simulink model "TVC_Model"  (R2019a)
settings: Solver=FixedStepAuto  StartTime=0.0  StopTime=ENV.t_f  FixedStep=.01  MaxStep=.01  RelTol=1e-3  EnableMultiTasking=on
undefined symbols (not defined in the file or in its folder): ACT, CTRL, ENV, Motor, VEH
libraries: Force_Moment_Sublibrary x4, Rail_UL x1, Environment_UL x1, Launch_Vehicle_CL x1
settings Model: ExtModeTrigDuration=2  Creator=John Jr  LastModifiedBy=John Jr
settings SolverCC: MaxConsecutiveMinStep=5
settings DataIOCC: LimitDataPoints=on  SaveFinalState=on  ReturnWorkspaceOutputs=off
settings OptimizationCC: DefaultParameterBehavior=Inlined  MaxStackSize=64
settings DebuggingCC: AllowSymbolicDim=off  SFUnexpectedBacktrackingDiag=warning  SFNoUnconditionalDefaultTransitionDiag=warning  SFExecutionAtInitializationDiag=none  ArithmeticOperatorsInVariantConditions=warning
settings HardwareCC: ProdBitPerInt=16  ProdBitPerPointer=16  ProdBitPerSizeT=16  ProdBitPerPtrDiffT=16  ProdLargestAtomicFloat=None  ProdWordSize=8  ProdHWDeviceType=Atmel->AVR  UseEmbeddedCoderFeatures=off  UseSimulinkCoderFeatures=off
settings ModelReferenceCC: PropagateSignalLabelsOutOfModel=off
settings SFSimCC: SimUseLocalCustomCode=off  MATLABDynamicMemAlloc=off
settings RTWCC: Description=Generic Real-Time Target  RTWUseLocalCustomCode=off  Toolchain=Microsoft Visual C++ 2019 v16.0 | nmake (64-bit Windows)  BuildConfiguration=Faster Runs
settings CodeAppCC: StateflowObjectComments=on
settings GRTTargetCC: TargetLangStandard=C89/C90 (ANSI)
settings ConfigComp: CovMetricSettings=dw  CovHtmlReporting=on  CovSaveCumulativeToWorkspaceVar=on  CovSaveSingleToWorkspaceVar=on  CovExternalEMLEnable=off

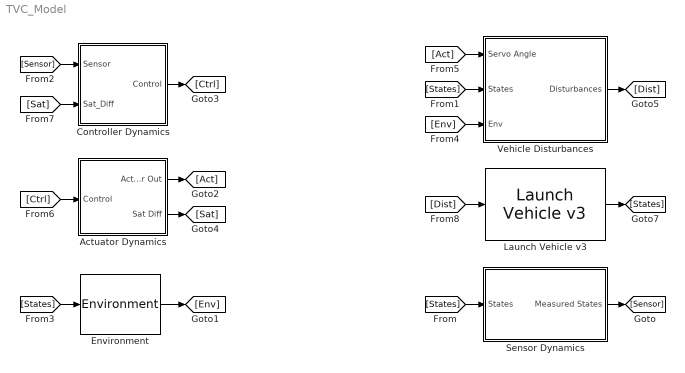
== system TVC_Model ==
  Actuator Dynamics : Subsystem
  Controller Dynamics : Subsystem
  Environment : Environment_UL/Environment  g=ENV.g  rho_b=ENV.rho_b  z_0=ENV.z_0  T=ENV.T  M=ENV.M  R=ENV.R  v_w0=ENV.v_w0  v_wf=ENV.v_wf
  Launch Vehicle v3 : Launch_Vehicle_CL/Launch Vehicle v3  SystemSampleTime=-1
  Sensor Dynamics : Subsystem
  Vehicle Disturbances : Subsystem
  wires:
  Launch Vehicle v3/1 -> [States]
  [States] -> Sensor Dynamics/1(States)
  [States] -> Vehicle Disturbances/2(States)
  Sensor Dynamics/1(Measured States) -> [Sensor]
  [Sensor] -> Controller Dynamics/1(Sensor)
  [States] -> Environment/1
  Environment/1 -> [Env]
  [Env] -> Vehicle Disturbances/3(Env)
  Actuator Dynamics/1(Actuator Out) -> [Act]
  [Act] -> Vehicle Disturbances/1(Servo Angle)
  Controller Dynamics/1(Control) -> [Ctrl]
  [Ctrl] -> Actuator Dynamics/1(Control)
  Actuator Dynamics/2(Sat Diff) -> [Sat]
  [Sat] -> Controller Dynamics/2(Sat_Diff)
  Vehicle Disturbances/1(Disturbances) -> [Dist]
  [Dist] -> Launch Vehicle v3/1

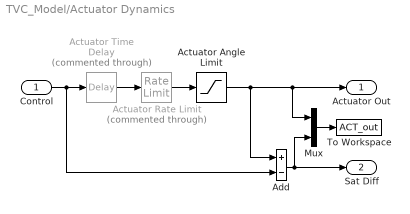
== system TVC_Model/Actuator Dynamics ==
  Control : Inport
  Actuator Angle Limit : Saturate  UpperLimit=ACT.u_max  LowerLimit=ACT.u_min
  Actuator Rate Limit : RateLimiter  Commented=through  RisingSlewLimit=ACT.w_s  FallingSlewLimit=-ACT.w_s  SampleTimeMode=inherited
  Actuator Time Delay : TransportDelay  Commented=through  DelayTime=ACT.tau
  Add : Sum  Inputs=+-
  Mux : Mux  Inputs=2
  To Workspace : ToWorkspace  VariableName=ACT_out  SaveFormat=Structure With Time  SampleTime=-1
  Actuator Out : Outport
  Sat Diff : Outport  Port=2
  wires:
  Actuator Rate Limit/1 -> Actuator Angle Limit/1
  Control/1 -> Add/2, Actuator Time Delay/1
  Add/1 -> Sat Diff/1, Mux/2
  Actuator Angle Limit/1 -> Add/1, Actuator Out/1, Mux/1
  Actuator Time Delay/1 -> Actuator Rate Limit/1
  Mux/1 -> To Workspace/1

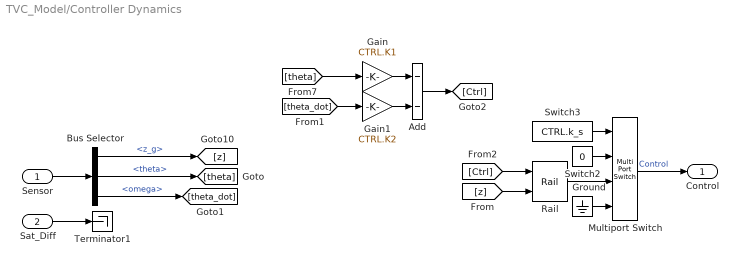
== system TVC_Model/Controller Dynamics ==
  Sensor : Inport
  Sat_Diff : Inport  Port=2
  Add : Sum  Inputs=--
  Bus Selector : BusSelector  OutputSignals=z_g,theta,omega
  Gain : Gain  Gain=CTRL.K1
  Gain1 : Gain  Gain=CTRL.K2
  Ground : Ground
  Multiport Switch : MultiPortSwitch
  Rail : Rail_UL/Rail  z_r=ENV.z_r  t_b=Motor.t_b  a_out=0
  Switch2 : Constant  Value=0
  Switch3 : Constant  Value=CTRL.k_s
  Terminator1 : Terminator
  Control : Outport
  wires:
  Switch3/1 -> Multiport Switch/1
  Switch2/1 -> Multiport Switch/2
  Sensor/1 -> Bus Selector/1
  Sat_Diff/1 -> Terminator1/1
  Bus Selector/2 -> [theta]  "<theta>"
  Bus Selector/3 -> [theta_dot]  "<omega>"
  Bus Selector/1 -> [z]  "<z_g>"
  [z] -> Rail/2
  Rail/1 -> Multiport Switch/3
  [Ctrl] -> Rail/1
  Add/1 -> [Ctrl]
  Gain/1 -> Add/1
  Gain1/1 -> Add/2
  [theta_dot] -> Gain1/1
  [theta] -> Gain/1
  Multiport Switch/1 -> Control/1  "Control"
  Ground/1 -> Multiport Switch/4

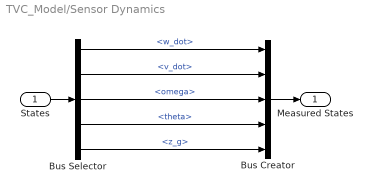
== system TVC_Model/Sensor Dynamics ==
  States : Inport
  Bus Creator : BusCreator  Inputs=5
  Bus Selector : BusSelector  OutputSignals=V_b_dot.w_dot,V_b_dot.v_dot,rot.omega,rot.theta,X_g.z_g
  Measured States : Outport
  wires:
  States/1 -> Bus Selector/1
  Bus Creator/1 -> Measured States/1
  Bus Selector/1 -> Bus Creator/1  "<w_dot>"
  Bus Selector/2 -> Bus Creator/2  "<v_dot>"
  Bus Selector/3 -> Bus Creator/3  "<omega>"
  Bus Selector/4 -> Bus Creator/4  "<theta>"
  Bus Selector/5 -> Bus Creator/5  "<z_g>"

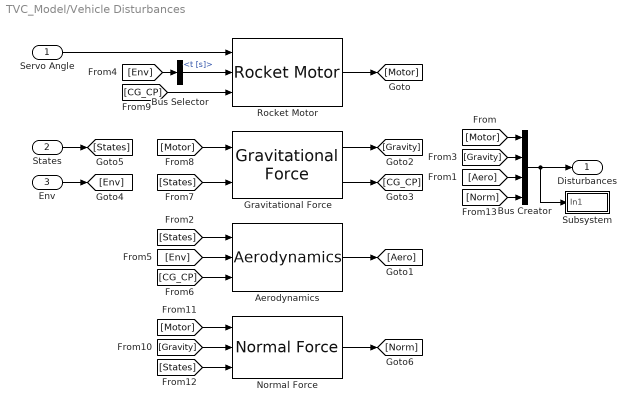
== system TVC_Model/Vehicle Disturbances ==
  Servo Angle : Inport
  States : Inport  Port=2
  Env : Inport  Port=3
  Aerodynamics : Force_Moment_Sublibrary/Aerodynamics  C_d=VEH.C_d  A_ref=VEH.A_ref  C_s=VEH.C_s  A_side=VEH.A_side  z_r=0
  Bus Creator : BusCreator  Inputs=4
  Bus Selector : BusSelector  OutputSignals=t [s]
  Gravitational Force : Force_Moment_Sublibrary/Gravitational Force  g=ENV.g  m=VEH.m  J=VEH.J  CG1=VEH.CG_1  CG2=VEH.CG_2  CP=VEH.CP  t_b=Motor.t_b
  Normal Force : Force_Moment_Sublibrary/Normal Force  SystemSampleTime=-1
  Rocket Motor : Force_Moment_Sublibrary/Rocket Motor  F_th=Motor.F_th  t_vec=Motor.T_b  t_b=Motor.t_b  m_m=Motor.m_m  m_f=Motor.m_f  k=Motor.k_m  L=VEH.L
  Subsystem : Subsystem
      mask Display:
      | patch([0 1 1 0], [0 0 1 1],[.8 1 .8])
      | 
      | 
      | 
      | disp('Log','texmode','on')
  Disturbances : Outport
  wires:
  Bus Creator/1 -> Subsystem/1(In1), Disturbances/1
  Rocket Motor/1 -> [Motor]
  States/1 -> [States]
  Servo Angle/1 -> Rocket Motor/1
  Env/1 -> [Env]
  [Env] -> Bus Selector/1
  Bus Selector/1 -> Rocket Motor/2  "<t [s]>"
  [Aero] -> Bus Creator/3
  [Motor] -> Bus Creator/1
  Aerodynamics/1 -> [Aero]
  [States] -> Aerodynamics/1
  [Env] -> Aerodynamics/2
  [CG_CP] -> Aerodynamics/3
  [States] -> Gravitational Force/2
  [Motor] -> Gravitational Force/1
  Gravitational Force/1 -> [Gravity]
  Gravitational Force/2 -> [CG_CP]
  [CG_CP] -> Rocket Motor/3
  [Gravity] -> Normal Force/2
  [Motor] -> Normal Force/1
  Normal Force/1 -> [Norm]
  [States] -> Normal Force/3
  [Gravity] -> Bus Creator/2
  [Norm] -> Bus Creator/4

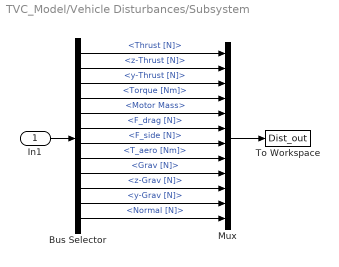
== system TVC_Model/Vehicle Disturbances/Subsystem ==
  In1 : Inport
  Bus Selector : BusSelector  OutputSignals=Motor.Thrust [N],Motor.z-Thrust [N],Motor.y-Thrust [N],Motor.Torque [Nm],Motor.Motor Mass,Aerodynamics.F_drag [N],Aerodynamics.F_side [N],Aerodynamics.T_aero [Nm],Gravity.Grav [N],Gravity.z-Grav [N],Gravity.y-Grav [N],Normal [N]
  Mux : Mux  Inputs=12
  To Workspace : ToWorkspace  VariableName=Dist_out  SaveFormat=Structure With Time  SampleTime=-1
  wires:
  In1/1 -> Bus Selector/1
  Mux/1 -> To Workspace/1
  Bus Selector/1 -> Mux/1  "<Thrust [N]>"
  Bus Selector/2 -> Mux/2  "<z-Thrust [N]>"
  Bus Selector/3 -> Mux/3  "<y-Thrust [N]>"
  Bus Selector/4 -> Mux/4  "<Torque [Nm]>"
  Bus Selector/5 -> Mux/5  "<Motor Mass>"
  Bus Selector/6 -> Mux/6  "<F_drag [N]>"
  Bus Selector/7 -> Mux/7  "<F_side [N]>"
  Bus Selector/8 -> Mux/8  "<T_aero [Nm]>"
  Bus Selector/9 -> Mux/9  "<Grav [N]>"
  Bus Selector/10 -> Mux/10  "<z-Grav [N]>"
  Bus Selector/11 -> Mux/11  "<y-Grav [N]>"
  Bus Selector/12 -> Mux/12  "<Normal [N]>"
